simulink model "ShootingControlSystem_working"  (R2024b)
settings: Solver=VariableStepAuto  StartTime=0.0  StopTime=10.0  RelTol=1e-3
libraries: slpidlib x2
settings Model: Creator=Dell  LastModifiedBy=Dell

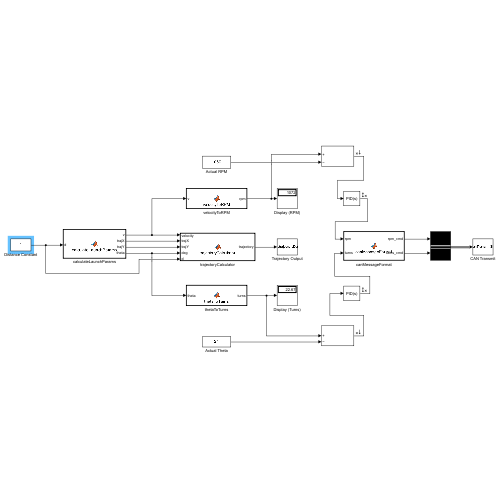
[thumbnail: Simulink's stored preview of the top-level diagram]
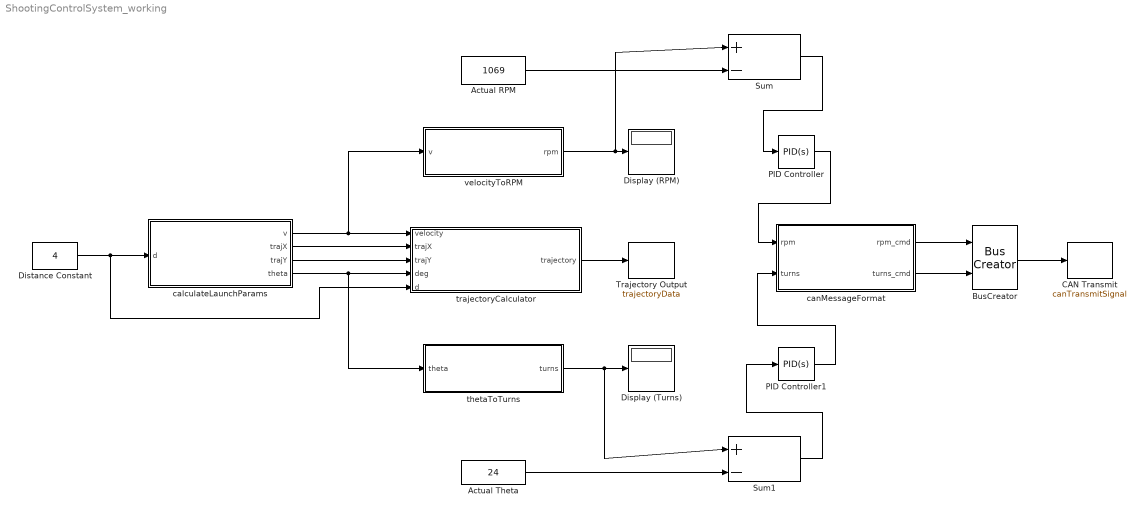
== system ShootingControlSystem_working ==
  Actual RPM : Constant  Value=1069
  Actual Theta : Constant  Value=24
  BusCreator : BusCreator  Inputs=2
  CAN Transmit : ToWorkspace  VariableName=canTransmitSignal  SaveFormat=Timeseries  SampleTime=-1
  Display (RPM) : Display
  Display (Turns) : Display
  Distance Constant : Constant  Value=4
  PID Controller : slpidlib/PID Controller  Controller=PID  Form=Parallel  TimeDomain=Continuous-time  UseExternalTs=off  SampleTime=-1  IntegratorMethod=Forward Euler  FilterMethod=Forward Euler  ControllerParametersSource=internal  P=0.5  I=-1  UseKiTs=off  D=0  UseExternalDerivativeSource=off  N=100  UseFilter=on  TunerSelectOption=Transfer Function Based (PID Tuner App)  InitialConditionSource=internal  InitialConditionForIntegrator=0  InitialConditionForFilter=0  DifferentiatorICPrevScaledInput=0  ExternalReset=none  TrackingMode=off  Kt=1  LimitOutput=off  SatLimitsSource=internal  UpperSaturationLimit=inf  LowerSaturationLimit=-inf  LinearizeAsGain=on  AntiWindupMode=none  Kb=1  LimitIntegrator=off  UpperIntegratorSaturationLimit=inf  LowerIntegratorSaturationLimit=-inf  POutMin=[]  POutMax=[]  IOutMin=[]  IOutMax=[]  DOutMin=[]  DOutMax=[]  NOutMin=[]  NOutMax=[]  SumOutMin=[]  SumOutMax=[]  SaturationOutMin=[]  SaturationOutMax=[]  PParamMin=[]  PParamMax=[]  IParamMin=[]  IParamMax=[]  DParamMin=[]  DParamMax=[]  NParamMin=[]  NParamMax=[]  KbParamMin=[]  KbParamMax=[]  KtParamMin=[]  KtParamMax=[]  KbOutMin=[]  KbOutMax=[]  KtOutMin=[]  KtOutMax=[]  IntegratorOutMin=[]  IntegratorOutMax=[]  FilterOutMin=[]  FilterOutMax=[]  SumI1OutMin=[]  SumI1OutMax=[]  SumI2OutMin=[]  SumI2OutMax=[]  SumI3OutMin=[]  SumI3OutMax=[]  SumI4OutMin=[]  SumI4OutMax=[]  SumDOutMin=[]  SumDOutMax=[]  DifferentiatorOutMin=[]  DifferentiatorOutMax=[]  FilterDiffOutCoefMin=[]  FilterDiffOutCoefMax=[]  ReciprocalOutMin=[]  ReciprocalOutMax=[]  SumDenOutMin=[]  SumDenOutMax=[]  SumNumOutMin=[]  SumNumOutMax=[]  DivideOutMin=[]  DivideOutMax=[]  UdiffTsProdOutMin=[]  UdiffTsProdOutMax=[]  NTsProdOutMin=[]  NTsProdOutMax=[]  UintegralTsProdOutMin=[]  UintegralTsProdOutMax=[]  UngainTsProdOutMin=[]  UngainTsProdOutMax=[]  ClampingZeroOutDataTypeStr=Inherit: Inherit via back propagation  ClampingZeroOutMin=[]  ClampingZeroOutMax=[]  FilterDenConstantOutDataTypeStr=Inherit: Inherit via back propagation  FilterDenConstantOutMin=[]  FilterDenConstantOutMax=[]  PCopyOutDataTypeStr=Inherit: Inherit via back propagation  PCopyOutMin=[]  PCopyOutMax=[]  NCopyOutDataTypeStr=Inherit: Inherit via back propagation  NCopyOutMin=[]  NCopyOutMax=[]  IntegratorContinuousStateAttributes=''  IntegratorStateMustResolveToSignalObject=off  IntegratorRTWStateStorageClass=Auto  FilterContinuousStateAttributes=''  FilterStateMustResolveToSignalObject=off  FilterRTWStateStorageClass=Auto  ParallelPVariant=InternalParameters  IdealPVariant=Disabled  IVariant=InternalParameters  DVariant=InternalParameters  IntegratorVariant=Continuous  SatVariant=Disabled  AWVariant=Passthrough  PCopyVariant=Disabled  TRVariant=Disabled  FdbkBlocksVariant=Forward  IdealPFdbkVariant=Disabled  SatFdbkVariant=Disabled  DerivativeFilterVariant=ContFilter  NVariant=InternalParameters  NCopyVariant=Disabled  FilterICVariant=InternalICsFilter  IntegratorICVariant=InternalICs  ExternalResetVariant=Disabled  TRSumVariant=Passthrough  SumFdbkVariant=Disabled  SumVariant=Sum_PID  TsampFilterVariant=InternalTs  TsampNgainVariant=Passthrough  TsampIntegralVariant=Disabled_SignalSpec  ExternalSaturationOutDataTypeStr=Inherit: Same as second input  DerivativeSourceVariant=ErrorSignal  PreIntVariant=InternalPreInt
  PID Controller1 : slpidlib/PID Controller  Controller=PID  Form=Parallel  TimeDomain=Continuous-time  UseExternalTs=off  SampleTime=-1  IntegratorMethod=Forward Euler  FilterMethod=Forward Euler  ControllerParametersSource=internal  P=1  I=1  UseKiTs=off  D=0  UseExternalDerivativeSource=off  N=100  UseFilter=on  TunerSelectOption=Transfer Function Based (PID Tuner App)  InitialConditionSource=internal  InitialConditionForIntegrator=0  InitialConditionForFilter=0  DifferentiatorICPrevScaledInput=0  ExternalReset=none  TrackingMode=off  Kt=1  LimitOutput=off  SatLimitsSource=internal  UpperSaturationLimit=inf  LowerSaturationLimit=-inf  LinearizeAsGain=on  AntiWindupMode=none  Kb=1  LimitIntegrator=off  UpperIntegratorSaturationLimit=inf  LowerIntegratorSaturationLimit=-inf  POutMin=[]  POutMax=[]  IOutMin=[]  IOutMax=[]  DOutMin=[]  DOutMax=[]  NOutMin=[]  NOutMax=[]  SumOutMin=[]  SumOutMax=[]  SaturationOutMin=[]  SaturationOutMax=[]  PParamMin=[]  PParamMax=[]  IParamMin=[]  IParamMax=[]  DParamMin=[]  DParamMax=[]  NParamMin=[]  NParamMax=[]  KbParamMin=[]  KbParamMax=[]  KtParamMin=[]  KtParamMax=[]  KbOutMin=[]  KbOutMax=[]  KtOutMin=[]  KtOutMax=[]  IntegratorOutMin=[]  IntegratorOutMax=[]  FilterOutMin=[]  FilterOutMax=[]  SumI1OutMin=[]  SumI1OutMax=[]  SumI2OutMin=[]  SumI2OutMax=[]  SumI3OutMin=[]  SumI3OutMax=[]  SumI4OutMin=[]  SumI4OutMax=[]  SumDOutMin=[]  SumDOutMax=[]  DifferentiatorOutMin=[]  DifferentiatorOutMax=[]  FilterDiffOutCoefMin=[]  FilterDiffOutCoefMax=[]  ReciprocalOutMin=[]  ReciprocalOutMax=[]  SumDenOutMin=[]  SumDenOutMax=[]  SumNumOutMin=[]  SumNumOutMax=[]  DivideOutMin=[]  DivideOutMax=[]  UdiffTsProdOutMin=[]  UdiffTsProdOutMax=[]  NTsProdOutMin=[]  NTsProdOutMax=[]  UintegralTsProdOutMin=[]  UintegralTsProdOutMax=[]  UngainTsProdOutMin=[]  UngainTsProdOutMax=[]  ClampingZeroOutDataTypeStr=Inherit: Inherit via back propagation  ClampingZeroOutMin=[]  ClampingZeroOutMax=[]  FilterDenConstantOutDataTypeStr=Inherit: Inherit via back propagation  FilterDenConstantOutMin=[]  FilterDenConstantOutMax=[]  PCopyOutDataTypeStr=Inherit: Inherit via back propagation  PCopyOutMin=[]  PCopyOutMax=[]  NCopyOutDataTypeStr=Inherit: Inherit via back propagation  NCopyOutMin=[]  NCopyOutMax=[]  IntegratorContinuousStateAttributes=''  IntegratorStateMustResolveToSignalObject=off  IntegratorRTWStateStorageClass=Auto  FilterContinuousStateAttributes=''  FilterStateMustResolveToSignalObject=off  FilterRTWStateStorageClass=Auto  ParallelPVariant=InternalParameters  IdealPVariant=Disabled  IVariant=InternalParameters  DVariant=InternalParameters  IntegratorVariant=Continuous  SatVariant=Disabled  AWVariant=Passthrough  PCopyVariant=Disabled  TRVariant=Disabled  FdbkBlocksVariant=Forward  IdealPFdbkVariant=Disabled  SatFdbkVariant=Disabled  DerivativeFilterVariant=ContFilter  NVariant=InternalParameters  NCopyVariant=Disabled  FilterICVariant=InternalICsFilter  IntegratorICVariant=InternalICs  ExternalResetVariant=Disabled  TRSumVariant=Passthrough  SumFdbkVariant=Disabled  SumVariant=Sum_PID  TsampFilterVariant=InternalTs  TsampNgainVariant=Passthrough  TsampIntegralVariant=Disabled_SignalSpec  ExternalSaturationOutDataTypeStr=Inherit: Same as second input  DerivativeSourceVariant=ErrorSignal  PreIntVariant=InternalPreInt
  Sum : Sum  Inputs=|+|-
  Sum1 : Sum  Inputs=|+-
  Trajectory Output : ToWorkspace  VariableName=trajectoryData  SaveFormat=Timeseries  SampleTime=-1
  calculateLaunchParams : MATLAB Function  TreatAsAtomicUnit=on
  canMessageFormat : MATLAB Function  TreatAsAtomicUnit=on
  thetaToTurns : MATLAB Function  TreatAsAtomicUnit=on
  trajectoryCalculator : MATLAB Function  TreatAsAtomicUnit=on
  velocityToRPM : MATLAB Function  TreatAsAtomicUnit=on
  wires:
  Distance Constant/1 -> trajectoryCalculator/5(d), calculateLaunchParams/1(d)
  calculateLaunchParams/1(v) -> velocityToRPM/1(v), trajectoryCalculator/1(velocity)
  canMessageFormat/1(rpm_cmd) -> BusCreator/1
  BusCreator/1 -> CAN Transmit/1
  trajectoryCalculator/1(trajectory) -> Trajectory Output/1
  canMessageFormat/2(turns_cmd) -> BusCreator/2
  calculateLaunchParams/4(theta) -> thetaToTurns/1(theta), trajectoryCalculator/4(deg)
  calculateLaunchParams/3(trajY) -> trajectoryCalculator/3(trajY)
  calculateLaunchParams/2(trajX) -> trajectoryCalculator/2(trajX)
  velocityToRPM/1(rpm) -> Sum/1, Display (RPM)/1
  thetaToTurns/1(turns) -> Sum1/1, Display (Turns)/1
  PID Controller1/1 -> canMessageFormat/2(turns)
  Actual RPM/1 -> Sum/2
  Actual Theta/1 -> Sum1/2
  Sum/1 -> PID Controller/1
  Sum1/1 -> PID Controller1/1
  PID Controller/1 -> canMessageFormat/1(rpm)

== matlab function ShootingControlSystem_working/velocityToRPM ==
  data: v input; rpm output
function rpm = velocityToRPM(v)

if v <= 0
    rpm = 0;
    return;
end

pulley_radius = 0.075; 
linear_per_rotation = 2 * pi * pulley_radius; 

rps = v / linear_per_rotation; 
rpm = rps * 60; 
end

== matlab function ShootingControlSystem_working/calculateLaunchParams ==
  data: d input; v output; trajX output; trajY output; theta output
function [v, trajX, trajY, theta] = calculateLaunchParams(d)

g = 9.81;
h0 = 1.46;  
hf = 2.43;  
hoop_distance = d; 

trajX = zeros(1, 5000); 
trajY = zeros(1, 5000);

theta = 70;  
best_angle = -1;
best_velocity = -1;
best_trajX = zeros(1, 5000);
best_trajY = zeros(1, 5000);
best_trajIdx = 0; 

while theta >= 50
    lower_vel = 5.0;
    upper_vel = 8.5;
    while upper_vel - lower_vel > 0.05
        mid_vel = (lower_vel + upper_vel) * 0.5;

        [success, tempX, tempY, tempIdx] = simulateProjectileMotion(theta, mid_vel, hoop_distance, hf, h0);

        if success
            best_velocity = mid_vel;
            best_angle = theta;
            best_trajX = tempX;
            best_trajY = tempY;
            best_trajIdx = tempIdx;
            upper_vel = mid_vel;
        else
            lower_vel = mid_vel;
        end
    end

    if best_velocity > 0
        break;
    end
    theta = theta - 1;
end

if best_velocity <= 0
    v = calculateVelocityForShot(hoop_distance, hf, h0);  
    theta = 60;  
    
    g = 9.81;         
    h0 = 1.46;         
    
    thetaRad = deg2rad(theta);
    vx = v * cos(thetaRad);
    vy = v * sin(thetaRad);
    
    dt = 0.01;
    maxT = 2;  
    numPoints = min(5000, ceil(maxT/dt));
    
    trajX = zeros(1, 5000);
    trajY = zeros(1, 5000);
    
    for i = 1:numPoints
        t = (i-1) * dt;
        trajX(i) = vx * t;
        trajY(i) = h0 + vy * t - 0.5 * g * t^2;
        
        if trajY(i) < 0
            trajY(i) = 0;
            break;
        end
    end
else
    v = best_velocity;
    theta = best_angle;
    trajX = best_trajX;
    trajY = best_trajY;
    
    if best_trajIdx < 5000
        trajX((best_trajIdx+1):end) = 0;
        trajY((best_trajIdx+1):end) = 0;
    end
end

end


function v = calculateVelocityForShot(target_distance, target_height, release_height)

g = 9.81;  
theta = 60; 

thetaRad = deg2rad(theta);

v = sqrt((g * target_distance^2) / (2 * cos(thetaRad)^2 * (target_distance * tan(thetaRad) - (target_height - release_height))));

end


function [success, xData, yData, trajIdx] = simulateProjectileMotion(angle, velocity, target_distance, target_height, release_height)

g = 9.81;
air_density = 1.225;
drag_coeff = 0.54;
ball_diameter = 0.239;
ball_mass = 0.6;

thetaRad = deg2rad(angle);
vx = velocity * cos(thetaRad);
vy = velocity * sin(thetaRad);

x = 0;
y = release_height;
dt = 0.01;
cross_sectional_area = pi * (ball_diameter / 2)^2;

xData = zeros(1, 5000);
yData = zeros(1, 5000);
trajIdx = 1;
success = false;

while y >= 0 && x <= target_distance + 0.5 && trajIdx <= 5000
    xData(trajIdx) = x;
    yData(trajIdx) = y;

    speed = sqrt(vx^2 + vy^2);
    if speed < 1e-6
        return;
    end

    drag_force = 0.5 * air_density * cross_sectional_area * drag_coeff * speed^2;

    ax = (-drag_force * vx / speed) / ball_mass;
    ay = -g + (-drag_force * vy / speed) / ball_mass;

    vx = vx + ax * dt;
    vy = vy + ay * dt;
    x = x + vx * dt;
    y = y + vy * dt;

    if abs(x - target_distance) < 0.05 && abs(y - target_height) < 0.05
        success = true;
        return;
    end

    dt = max(0.005, min(0.5 / speed, 0.01)); 
    trajIdx = trajIdx + 1;
end

end

== matlab function ShootingControlSystem_working/thetaToTurns ==
  data: theta input; turns output
function turns = thetaToTurns(theta)

if theta <= 0
    turns = 0;
    return;
end

total_pitch_range = 30; 
lead_screw_total_turns = 10; 

turns = (theta / total_pitch_range) * lead_screw_total_turns;
end

== matlab function ShootingControlSystem_working/canMessageFormat ==
  data: rpm input; rpm_cmd output; turns input; turns_cmd output
function [rpm_cmd, turns_cmd] = canMessageFormat(rpm, turns)

    assert(isnumeric(rpm) && isscalar(rpm), 'rpm should be a numeric scalar');
    assert(isnumeric(turns) && isscalar(turns), 'turns should be a numeric scalar');
    
    rpm_cmd = rpm;
    turns_cmd = turns;
end

== matlab function ShootingControlSystem_working/trajectoryCalculator ==
  data: velocity input; trajX input; trajY input; trajectory output; deg input; d input
function trajectory = trajectoryCalculator(velocity, trajX, trajY, deg, d)

trajectory = zeros(2, 5000);


validIdx = trajX > 0 | trajY > 0;

validX = trajX(validIdx);
validY = trajY(validIdx);

if ~isempty(validX)
    numPoints = min(length(validX), 5000);
    trajectory(1, 1:numPoints) = validX(1:numPoints);
    trajectory(2, 1:numPoints) = validY(1:numPoints);
else
   
    g = 9.81; 
    initialHeight = 1.43;
    
    angle_rad = deg * pi / 180;
    
    vx = velocity * cos(angle_rad);
    vy = velocity * sin(angle_rad);
    
    N = 100;
    t_hoop = d / vx;
    t = linspace(0, t_hoop, N);
    
    x = vx * t;
    y = initialHeight + vy * t - 0.5 * g * t.^2;
    
    y(y < 0) = 0;
    
    trajectory(1, 1:N) = x;
    trajectory(2, 1:N) = y;
end
end
